simulink model "tendons_simulink"  (R2026a)
settings: Solver=ode4  FixedStep=pp.Ts_plant
values from neighbouring files (symbols this model uses):
  params =     [CEM_no_singularity_animation_data.mat]    (also in CEM_singularity_animation_data.mat; test_mpc_singularity_warning_sweep.m = baseParams)
undefined symbols (not defined in the file or in its folder): pp
settings Model: Creator=ryanj  LastModifiedBy=SWP
settings DataIOCC: InspectSignalLogs=on

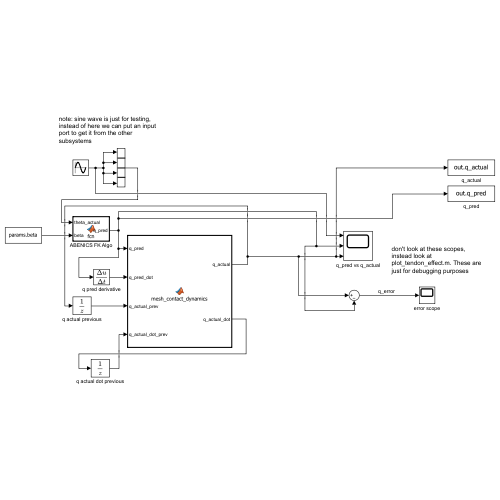
[thumbnail: Simulink's stored preview of the top-level diagram]
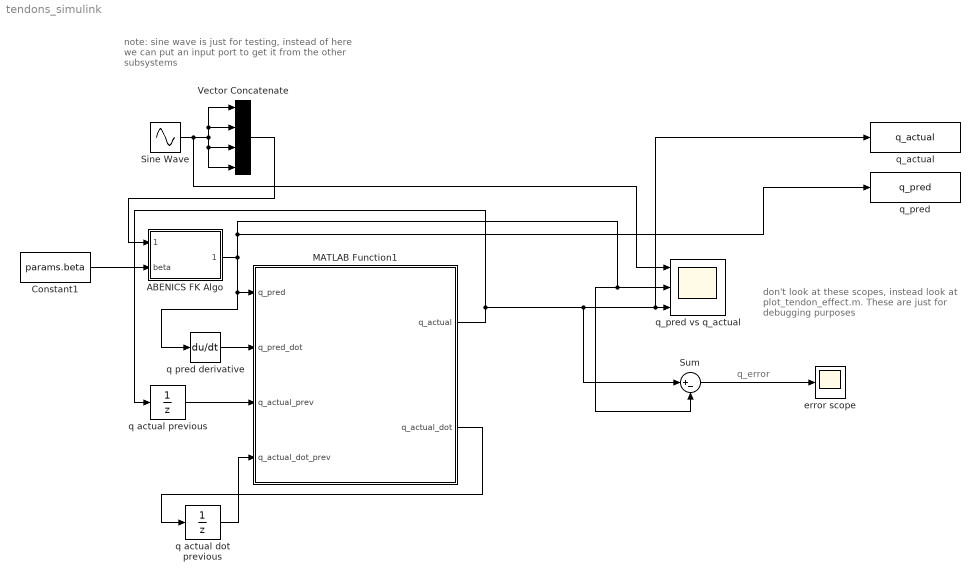
== system tendons_simulink ==
  note: don't look at these scopes, instead look at plot_tendon_effect.m. These are just for debugging purposes
  note: note: sine wave is just for testing, instead of here we can put an input port to get it from the other subsystems
  note: q_error
  ABENICS FK Algo : MATLAB Function  TreatAsAtomicUnit=on
  Constant1 : Constant  Value=params.beta  SampleTime=params.Ts
  MATLAB Function1 : MATLAB Function  TreatAsAtomicUnit=on
  Sine Wave : Sin  SampleTime=0
  Sum : Sum  Inputs=|+-
  Vector Concatenate : Concatenate  NumInputs=4
  error scope : Scope
      settings: ActiveDisplayYMinimum=-0.060487454138757064  ActiveDisplayYMaximum=0.053081000942398475
  q actual dot previous : UnitDelay  InitialCondition=[0; 0; 0]  SampleTime=pp.Ts_plant
  q actual previous : UnitDelay  InitialCondition=[0; 0; 0]  SampleTime=pp.Ts_plant
  q pred derivative : Derivative
  q_actual : ToWorkspace  VariableName=q_actual  SaveFormat=Timeseries  SampleTime=-1
  q_pred : ToWorkspace  VariableName=q_pred  SaveFormat=Timeseries  SampleTime=-1
  q_pred vs q_actual : Scope  NumInputPorts=3
      settings: Title=Backlash  ActiveDisplayYMinimum=-1.2357133279335126  ActiveDisplayYMaximum=1.8136071169829846
  wires:
  ABENICS FK Algo/1(q_pred) -> q pred derivative/1, MATLAB Function1/1(q_pred), q_pred vs q_actual/2, Sum/2, q_pred/1
  MATLAB Function1/1(q_actual) -> q_actual/1, q_pred vs q_actual/3, Sum/1, q actual previous/1
  Sine Wave/1 -> q_pred vs q_actual/1, Vector Concatenate/2, Vector Concatenate/1, Vector Concatenate/4, Vector Concatenate/3
  Vector Concatenate/1 -> ABENICS FK Algo/1(theta_actual)
  MATLAB Function1/2(q_actual_dot) -> q actual dot previous/1
  q actual previous/1 -> MATLAB Function1/3(q_actual_prev)
  q actual dot previous/1 -> MATLAB Function1/4(q_actual_dot_prev)
  q pred derivative/1 -> MATLAB Function1/2(q_pred_dot)
  Sum/1 -> error scope/1
  Constant1/1 -> ABENICS FK Algo/2(beta)

== matlab function tendons_simulink/ABENICS FK Algo ==
  data: theta_actual input size=[4,1]; q_pred output size=[3,1]; beta input
function q_pred = fcn(theta_actual, beta)
%#codegen

params.beta = beta;
q_pred = abenicsFK(theta_actual, params);

end

function [q_pred, info] = abenicsFK(theta_actual, params)
%abenicsFK Analytic 4-input FK for ABENICS orientation prediction.
%
% Input:
%   theta_actual = [theta_rA; theta_pA; theta_rB; theta_pB] in radians
%   params       = ABENICS parameter structure with params.beta
%
% Output:
%   q_pred       = [roll; pitch; yaw] in radians
%   info         = diagnostic structure
%
% Project convention:
%   theta_actual is output-side MP gear angle, not raw motor shaft angle.
%
% Important:
%   This FK uses all four theta values.
%   It builds one CS-gear orientation axis from module A,
%   one CS-gear orientation axis from module B,
%   then uses a cross product to complete the rotation matrix.

    if ~isequal(size(theta_actual), [4, 1])
        error('abenicsFK:thetaSize', ...
              'theta_actual must be [theta_rA; theta_pA; theta_rB; theta_pB].');
    end

    if nargin < 2 || ~isfield(params, 'beta')
        error('abenicsFK:missingBeta', ...
              'params.beta is required.');
    end

    beta = params.beta;

    if ~isscalar(beta)
        error('abenicsFK:betaSize', ...
              'params.beta must be scalar.');
    end

    theta_rA = theta_actual(1);
    theta_pA = theta_actual(2);
    theta_rB = theta_actual(3);
    theta_pB = theta_actual(4);

    % Convert output-side MP gear angles to paper-style chain angles
    theta_A1 = theta_rA;
    theta_A2 = -0.5 * theta_pA;

    theta_B1 = theta_rB;
    theta_B2 = -0.5 * theta_pB;

    % -----------------------------
    % Module A axis contribution
    % -----------------------------
    c1 = [cos(theta_A2);
          sin(theta_A1) * sin(theta_A2);
         -cos(theta_A1) * sin(theta_A2)];

    % -----------------------------
    % Module B axis contribution
    %
    % This is the sign/order-sensitive part.
    % It must be verified by IK -> FK round-trip tests.
    % -----------------------------
    v2_B = [cos(theta_B2);
           -sin(theta_B1) * sin(theta_B2);
            cos(theta_B1) * sin(theta_B2)];

    c2 = localRz(beta) * v2_B;

    % -----------------------------
    % Diagnostics before cleanup
    % -----------------------------
    c1Norm = norm(c1);
    c2Norm = norm(c2);
    rawColumnDot = dot(c1, c2);
    rawCross = cross(c1, c2);
    rawCrossNorm = norm(rawCross);

    % -----------------------------
    % Orthonormalize columns
    %
    % e1 = cleaned first column
    % e2 = cleaned second column, made perpendicular to e1
    % e3 = e1 x e2
    % -----------------------------
    tol = 1e-12;

    if c1Norm < tol
        error('abenicsFK:c1Bad', ...
              'Module A column is near zero.');
    end

    e1 = c1 / c1Norm;

    c2_perp = c2 - dot(e1, c2) * e1;
    c2PerpNorm = norm(c2_perp);

    if c2PerpNorm < tol
        error('abenicsFK:columnsParallel', ...
              'Module A and B columns are nearly parallel. FK orientation is poorly defined.');
    end

    e2 = c2_perp / c2PerpNorm;

    e3 = cross(e1, e2);
    e3 = e3 / norm(e3);

    R_BH = [e1, e2, e3];

    % Convert rotation matrix into [roll; pitch; yaw]
    q_pred = localRotmToXYZEuler(R_BH);

    % -----------------------------
    % Diagnostics
    % -----------------------------
    info = struct();
    info.c1 = c1;
    info.c2 = c2;
    info.e1 = e1;
    info.e2 = e2;
    info.e3 = e3;
    info.R_BH = R_BH;

    info.c1Norm = c1Norm;
    info.c2Norm = c2Norm;
    info.columnDot = rawColumnDot;
    info.crossNorm = rawCrossNorm;
    info.c2PerpNorm = c2PerpNorm;
    info.detR = det(R_BH);

    % Useful singularity-ish clue:
    % small means the two module-defined axes are almost parallel
    info.columnSeparationScore = rawCrossNorm;

    if rawCrossNorm < 1e-6
        warning('abenicsFK:nearParallelColumns', ...
                'Module A and B columns are nearly parallel. This may indicate a singular or poorly conditioned configuration.');
    end

    if ~isequal(size(q_pred), [3, 1])
        error('abenicsFK:qPredSize', ...
              'q_pred must be 3x1.');
    end
end

function R = localRz(theta)
    c = cos(theta);
    s = sin(theta);

    R = [c, -s, 0;
         s,  c, 0;
         0,  0, 1];
end

function x_clamped = localClamp(x, lower, upper)
    x_clamped = min(upper, max(lower, x));
end

function q = localRotmToXYZEuler(R)
% Uses convention:
%   R = Rx(roll) * Ry(pitch) * Rz(yaw)

    tol = 1e-12;

    pitch_arg = localClamp(R(1,3), -1, 1);
    pitch = asin(pitch_arg);

    cp = cos(pitch);

    if abs(cp) > tol
        roll = atan2(-R(2,3), R(3,3));
        yaw  = atan2(-R(1,2), R(1,1));
    else
        roll = 0;
        yaw  = atan2(R(2,1), R(2,2));
    end

    q = [roll;
         pitch;
         yaw];
end

== matlab function tendons_simulink/MATLAB Function1 ==
  data: q_pred input size=[3 1]; q_pred_dot input size=[3 1]; q_actual output size=[3 1]; q_actual_prev input size=[3 1]; q_actual_dot_prev input size=[3 1]; q_actual_dot output size=[3 1]; meshContact parameter
function [q_actual, q_actual_dot] = mesh_contact_dynamics( ...
                    q_pred, q_pred_dot, ...
                    q_actual_prev, q_actual_dot_prev, meshContact)
%#codegen
%
% Models backlash and compliant gear contact independently for
% roll, pitch, and yaw.
%
% Tendon preload reduces the effective backlash width:
%
%   effective_backlash = mesh_backlash - alpha_preload*tau_preload
%
% Preload is not added directly to the net output torque.

    Ts = meshContact.Ts;

    % -------------------------------------------------------------
    % Preload-dependent effective backlash
    % -------------------------------------------------------------
    % Units:
    %   mesh_backlash   : rad
    %   tau_preload_mesh: N*m
    %   alpha_preload   : rad/(N*m)
    %
    % max(...,0) prevents preload from creating negative backlash.
    effective_backlash = max( ...
        meshContact.mesh_backlash ...
        - meshContact.alpha_preload .* abs(meshContact.tau_preload_mesh), ...
        zeros(3,1));

    half_bl = effective_backlash / 2;

    % Relative displacement and velocity between predicted and
    % actual motion.
    d     = q_actual_prev     - q_pred;
    d_dot = q_actual_dot_prev - q_pred_dot;

    % Inside the backlash region, there is no mesh stiffness.
    % Only a small free-motion damping force is present.
    Fc = -meshContact.c_free .* d_dot;

    % Apply the contact law independently to each rotational axis.
    for i = 1:3
        if d(i) > half_bl(i)

            % Contact with the positive side of the backlash gap.
            penetration = d(i) - half_bl(i);

            Fc(i) = -meshContact.k_mesh(i) * penetration ...
                    - meshContact.c_contact(i) * d_dot(i);

        elseif d(i) < -half_bl(i)

            % Contact with the negative side of the backlash gap.
            penetration = d(i) + half_bl(i);

            Fc(i) = -meshContact.k_mesh(i) * penetration ...
                    - meshContact.c_contact(i) * d_dot(i);
        end
    end

    % Gravity torque.
    tau_gravity = meshContact.tau_gravity_max ...
                  .* sin(q_actual_prev);

    % Preload is deliberately absent here. It changes engagement,
    % rather than acting as a driving torque.
    net = Fc - tau_gravity;

    % Integrate rotational dynamics.
    q_actual_dot = q_actual_dot_prev ...
                   + (net ./ meshContact.J_mesh) .* Ts;

    q_actual = q_actual_prev + q_actual_dot .* Ts;
end
